simulink model "PMSM_Control_Using_FOC_And_SVPWM_Conference"  (R2023b)
(part 2 of 5)

  Bus Selector15/2 -> Scope23/2  "<SOC (%)>"
  Bus Selector15/3 -> Scope23/3  "<Current (A)>"
  Signal Builder/1(torque) -> PMSM AC  5/1
  Speed_Path/1(speed) -> Sum18/1
  PID Controller22/1 -> PWM Generator (DC-DC)6/1
  Speed_Path1/1(speed) -> Sum29/1
  Signal Builder2/1(torque) -> PMSM AC  8/1
  SVPWM Generator (2-Level)8/1 -> Universal Bridge8/1
  PID Controller27/1 -> Scope25/1, Sum28/1
  Current Measurement2/1 -> Scope27/1
  Voltage Measurement8/1 -> Display13/1
  Gain23/1 -> Scope24/1
  Demux15/3 -> Terminator14/1
  Bus Selector17/6 -> Scope24/2  "<Electromagnetic torque Te (N*m)>"
  PID Controller29/1 -> Mux15/2
  PMSM AC  8/1 -> Bus Selector17/1
  Bus Selector17/3 -> Scope24/6, Mux16/3  "<Stator current is_c (A)>"
  Gain22/1 -> Sum29/2
  Sum27/1 -> Scope25/2, PID Controller28/1
  Bus Selector17/1 -> Scope24/4, Mux16/1  "<Stator current is_a (A)>"
  Constant36/1 -> Mux15/3
  PID Controller28/1 -> Mux15/1
  Mux15/1 -> dq0 to Alpha-Beta-Zero7/1
  Sum28/1 -> PID Controller29/1
  Bus Selector17/4 -> Gain23/1, Gain22/1  "<Rotor speed wm (rad/s)>"
  Demux16/2 -> Sum28/2
  Demux16/1 -> Sum27/2
  Bus Selector17/5 -> Scope24/3, Gain21/1  "<Rotor angle thetam (rad)>"
  Alpha-Beta-Zero to dq7/1 -> Demux16/1
  dq0 to Alpha-Beta-Zero7/1 -> Demux15/1
  Gain21/1 -> Alpha-Beta-Zero to dq7/2, dq0 to Alpha-Beta-Zero7/2
  Demux15/1 -> SVPWM Generator (2-Level)8/1
  Demux16/3 -> Terminator15/1
  Demux15/2 -> SVPWM Generator (2-Level)8/2
  Bus Selector17/2 -> Scope24/5, Mux16/2  "<Stator current is_b (A)>"
  Sum29/1 -> PID Controller27/1
  Constant34/1 -> Sum27/1
  abc to Alpha-Beta-Zero7/1 -> Alpha-Beta-Zero to dq7/1
  Voltage Measurement9/1 -> Display17/1, Sum31/2
  PWM Generator (DC-DC)4/1 -> Switch/3, Scope29/1
  Battery11/1 -> Bus Selector18/1
  Bus Selector18/1 -> Scope31/1  "<SOC (%)>"
  Step16/1 -> Add5/4
  Bus Selector18/3 -> Scope31/3  "<Voltage (V)>"
  Bus Selector18/2 -> Scope31/2  "<Current (A)>"
  Step13/1 -> Add5/1
  Current Measurement3/1 -> Sum30/2
  Step15/1 -> Add5/3
  Step14/1 -> Add5/2
  Voltage Measurement12/1 -> Display18/1
  Mux16/1 -> abc to Alpha-Beta-Zero7/1
  Add5/1 -> Sum30/1
  Sum30/1 -> PID Controller30/1
  PID Controller30/1 -> PWM Generator (DC-DC)4/1
  PID Controller31/1 -> PWM Generator (DC-DC)5/1
  Constant37/1 -> Sum31/1
  PWM Generator (DC-DC)5/1 -> Switch/1
  Sum31/1 -> PID Controller31/1
  Switch/1 -> Mosfet4/1, NOT/1
  NOT/1 -> Mosfet5/1
  Constant35/1 -> Switch/2
  Demux18/1 -> Sum32/2
  Battery8/1 -> Bus Selector19/1
  Demux18/3 -> Terminator17/1
  abc to Alpha-Beta-Zero8/1 -> Alpha-Beta-Zero to dq8/1
  Bus Selector16/2 -> Scope26/5, Mux18/2  "<Stator current is_b (A)>"
  PMSM AC  9/1 -> Bus Selector16/1
  Bus Selector16/4 -> Gain26/1, Gain25/1  "<Rotor speed wm (rad/s)>"
  Sum34/1 -> PID Controller32/1
  Speed_Path2/1(speed) -> Sum34/1
  PID Controller36/1 -> PWM Generator (DC-DC)9/1
  Signal Builder1/1(torque) -> PMSM AC  9/1
  Voltage Measurement14/1 -> Display14/1
  PID Controller33/1 -> Mux17/1
  Bus Selector16/1 -> Scope26/4, Mux18/1  "<Stator current is_a (A)>"
  SVPWM Generator (2-Level)9/1 -> Universal Bridge9/1
  Gain24/1 -> Alpha-Beta-Zero to dq8/2, dq0 to Alpha-Beta-Zero8/2
  Bus Selector16/3 -> Scope26/6, Mux18/3  "<Stator current is_c (A)>"
  Sum32/1 -> Scope28/2, PID Controller33/1
  Current Measurement4/1 -> Scope30/1
  Demux17/2 -> SVPWM Generator (2-Level)9/2
  Sum36/1 -> PID Controller36/1
  PID Controller32/1 -> Scope28/1, Sum33/1
  Gain26/1 -> Scope26/1
  PID Controller34/1 -> Mux17/2
  Bus Selector19/1 -> Scope32/1, Scope33/1  "<SOC (%)>"
  Demux17/1 -> SVPWM Generator (2-Level)9/1
  Constant40/1 -> Mux17/3
  Bus Selector19/3 -> Scope33/3  "<Voltage (V)>"
  Alpha-Beta-Zero to dq8/1 -> Demux18/1
  Bus Selector16/6 -> Scope32/2, Scope26/2  "<Electromagnetic torque Te (N*m)>"
  PWM Generator (DC-DC)9/1 -> Mosfet8/1, NOT1/1
  Sum33/1 -> PID Controller34/1
  Demux17/3 -> Terminator16/1
  Gain25/1 -> Sum34/2
  Demux18/2 -> Sum33/2
  Constant38/1 -> Sum32/1
  Mux18/1 -> abc to Alpha-Beta-Zero8/1
  Mux17/1 -> dq0 to Alpha-Beta-Zero8/1
  Bus Selector19/2 -> Scope33/2  "<Current (A)>"
  Bus Selector16/5 -> Scope26/3, Gain24/1  "<Rotor angle thetam (rad)>"
  dq0 to Alpha-Beta-Zero8/1 -> Demux17/1
  Voltage Measurement13/1 -> Display20/1
  NOT1/1 -> Mosfet9/1
  Constant41/1 -> Sum36/1
  Voltage Measurement15/1 -> Display19/1, Sum36/2
  Voltage Measurement18/1 -> Sum39/2, Display22/1
  Constant43/1 -> Sum39/1
  NOT2/1 -> Mosfet11/1
  Voltage Measurement16/1 -> Display23/1
  dq0 to Alpha-Beta-Zero9/1 -> Demux19/1
  Bus Selector20/5 -> Gain27/1, Scope34/3  "<Rotor angle thetam (rad)>"
  Bus Selector21/2 -> Scope38/2  "<Current (A)>"
  Mux19/1 -> dq0 to Alpha-Beta-Zero9/1
  Mux20/1 -> abc to Alpha-Beta-Zero9/1
  Constant39/1 -> Sum35/1
  Demux20/2 -> Sum37/2
  Gain28/1 -> Sum38/2
  Demux19/3 -> Terminator18/1
  Sum37/1 -> PID Controller38/1
  PWM Generator (DC-DC)8/1 -> NOT2/1, Mosfet10/1
  Bus Selector20/6 -> Scope34/2, Scope37/2  "<Electromagnetic torque Te (N*m)>"
  Alpha-Beta-Zero to dq9/1 -> Demux20/1
  Bus Selector21/3 -> Scope38/3  "<Voltage (V)>"
  Constant42/1 -> Mux19/3
  Demux19/1 -> SVPWM Generator (2-Level)10/1
  Bus Selector21/1 -> Scope38/1, Scope37/1  "<SOC (%)>"
  PID Controller38/1 -> Mux19/2
  Gain29/1 -> Scope34/1
  PID Controller35/1 -> Sum37/1, Scope35/1
  Sum39/1 -> PID Controller39/1
  Demux19/2 -> SVPWM Generator (2-Level)10/2
  Current Measurement6/1 -> Scope36/1
  Sum35/1 -> PID Controller37/1, Scope35/2
  Bus Selector20/3 -> Mux20/3, Scope34/6  "<Stator current is_c (A)>"
  Gain27/1 -> dq0 to Alpha-Beta-Zero9/2, Alpha-Beta-Zero to dq9/2
  SVPWM Generator (2-Level)10/1 -> Universal Bridge10/1
  Bus Selector20/1 -> Mux20/1, Scope34/4  "<Stator current is_a (A)>"
  PID Controller37/1 -> Mux19/1
  Voltage Measurement17/1 -> Display21/1
  Sum38/1 -> PID Controller35/1
  Bus Selector20/4 -> Gain28/1, Gain29/1  "<Rotor speed wm (rad/s)>"
  PMSM AC  10/1 -> Bus Selector20/1
  Bus Selector20/2 -> Mux20/2, Scope34/5  "<Stator current is_b (A)>"
  abc to Alpha-Beta-Zero9/1 -> Alpha-Beta-Zero to dq9/1
  Demux20/3 -> Terminator19/1
  Battery12/1 -> Bus Selector21/1
  Demux20/1 -> Sum35/2
  Multiport Switch/1 -> PMSM AC  10/1
  Scenario_Selection/1 -> Multiport Switch/1, Multiport Switch1/1
  Multiport Switch1/1 -> Sum38/1
  Speed_Path6/1(speed) -> Multiport Switch1/2
  Signal Builder8/1(torque) -> Multiport Switch/3
  Speed_Path8/1(speed) -> Multiport Switch1/3
  Demux22/1 -> Sum40/2
  PID Controller42/1 -> Mux21/2
  Bus Selector23/1 -> Scope43/1, Scope42/1  "<SOC (%)>"
  Bus Selector22/1 -> Mux22/1, Scope39/4  "<Stator current is_a (A)>"
  Bus Selector23/3 -> Scope43/3  "<Voltage (V)>"
  Bus Selector22/4 -> Gain31/1, Gain32/1  "<Rotor speed wm (rad/s)>"
  Demux21/2 -> SVPWM Generator (2-Level)11/2
  Sum42/1 -> PID Controller40/1
  Bus Selector22/6 -> Scope39/2  "<Electromagnetic torque Te (N*m)>"
  Switch2/1 -> Sum42/1
  Constant45/1 -> Mux21/3
  Bus Selector22/2 -> Mux22/2, Scope39/5  "<Stator current is_b (A)>"
  Gain30/1 -> dq0 to Alpha-Beta-Zero10/2, Alpha-Beta-Zero to dq10/2
  Demux22/3 -> Terminator21/1
  Demux22/2 -> Sum41/2
  Demux21/3 -> Terminator20/1
  SVPWM Generator (2-Level)11/1 -> Universal Bridge11/1
  Switch1/1 -> PMSM AC  11/1
  Sum41/1 -> PID Controller42/1
  Mux22/1 -> abc to Alpha-Beta-Zero10/1
  Scenario_Selection1/1 -> Switch2/2, Switch1/2
  Current Measurement8/1 -> Scope41/1
  Speed_Path3/1(speed) -> Switch2/1
  Sum40/1 -> PID Controller41/1, Scope40/2
  PID Controller41/1 -> Mux21/1
  Battery13/1 -> Bus Selector23/1
  PMSM AC  11/1 -> Bus Selector22/1
  Speed_Path5/1(speed) -> Switch2/3
  Signal Builder5/1(torque) -> Switch1/3
  Signal Builder3/1(torque) -> Switch1/1
  Mux21/1 -> dq0 to Alpha-Beta-Zero10/1
  Voltage Measurement19/1 -> Display26/1
  Gain32/1 -> Scope39/1
  PID Controller40/1 -> Sum41/1, Scope40/1
  dq0 to Alpha-Beta-Zero10/1 -> Demux21/1
  Voltage Measurement20/1 -> Display24/1
  Voltage Measurement21/1 -> Scope42/3, Display25/1
  Alpha-Beta-Zero to dq10/1 -> Demux22/1
  Demux21/1 -> SVPWM Generator (2-Level)11/1
  Gain31/1 -> Sum42/2
  Bus Selector23/2 -> Scope42/2, Scope43/2  "<Current (A)>"
  Constant44/1 -> Sum40/1
  abc to Alpha-Beta-Zero10/1 -> Alpha-Beta-Zero to dq10/1
  Bus Selector22/5 -> Gain30/1, Scope39/3  "<Rotor angle thetam (rad)>"
  Bus Selector22/3 -> Mux22/3, Scope39/6  "<Stator current is_c (A)>"
  Bus Selector24/1 -> Scope46/1, Display27/1  "<Voltage (V)>"
  Constant47/1 -> Sum44/2
  Battery14/1 -> Bus Selector24/1
  Bus Selector24/2 -> Display31/1, Scope46/2  "<Current (A)>"
  Bus Selector24/3 -> Scope46/3  "<SOC (%)>"
  PWM Generator (DC-DC)11/1 -> NOT4/1, Scope47/1, PWM_1/1
  NOT4/1 -> Scope48/1, PWM_2/1
  Current Measurement10/1 -> Display30/1
  Voltage Measurement23/1 -> Sum44/1, Scope45/1, Display28/1
  Voltage Measurement22/1 -> Display29/1
  From1/1 -> Mosfet14/1
  PID Controller45/1 -> PWM Generator (DC-DC)11/1, Display32/1
  Sum44/1 -> PID Controller45/1
  Constant48/1 -> Sum45/1
  Sum45/1 -> Fuzzy Logic Controller1/1
  Fuzzy Logic Controller1/1 -> Display33/1, PWM Generator (DC-DC)12/1
  NOT5/1 -> PWM_4/1, Scope50/1
  PWM Generator (DC-DC)12/1 -> PWM_3/1, Scope49/1, NOT5/1
  From/1 -> Mosfet15/1
  Voltage Measurement24/1 -> Scope51/1
  PWM Generator (DC-DC)13/1 -> Mosfet12/1, NOT6/1
  Constant50/1 -> PWM Generator (DC-DC)13/1
  PWM Generator (DC-DC)14/1 -> Mosfet16/1, NOT7/1
  NOT7/1 -> Mosfet17/1
  Constant51/1 -> PWM Generator (DC-DC)14/1
  NOT6/1 -> Mosfet13/1
  PID Controller39/1 -> PWM Generator (DC-DC)8/1
  PWM Generator (DC-DC)2/1 -> Mosfet3/1
  PWM Generator (DC-DC)3/1 -> Mosfet2/1
  Bus Selector25/2 -> Scope52/2, Scope44/2  "<Current (A)>"
  Voltage Measurement25/1 -> Display37/1
  Battery15/1 -> Bus Selector25/1
  Bus Selector25/3 -> Goto2/1, Scope52/3  "<Voltage (V)>"
  Bus Selector25/1 -> Scope44/1, Goto1/1, Scope52/1, Goto/1  "<SOC (%)>"
  From2/1 -> Mosfet22/1
  From3/1 -> Mosfet23/1
  Voltage Measurement27/1 -> Display38/1, Goto3/1
  Sum43/1 -> PID Controller43/1
  Constant53/1 -> Sum43/1
  From4/1 -> Sum43/2
  PID Controller43/1 -> Goto4/1
  PID Controller44/1 -> Gain33/1
  From5/1 -> Sum46/2
  Constant54/1 -> Sum46/1
  Sum46/1 -> PID Controller44/1
  Gain33/1 -> Goto5/1
  From6/1 -> Switch3/1
  From7/1 -> Switch3/3
  From8/1 -> Switch3/2
  Step10/1 -> Goto6/1
  From9/1 -> Ideal Switch/1
  From10/1 -> Sum47/2
  From11/1 -> Sum47/1
  Sum47/1 -> PID Controller46/1
  Switch3/1 -> Goto8/1
  PID Controller46/1 -> PWM Generator (DC-DC)16/1
  PWM Generator (DC-DC)16/1 -> NOT9/1, Goto7/1
  NOT9/1 -> Goto9/1
  From13/1 -> Mosfet19/1
  From12/1 -> Mosfet18/1
  Bus Selector26/1 -> Goto10/1, Scope54/1, Goto11/1, Scope53/1  "<SOC (%)>"
  Bus Selector26/3 -> Scope54/3, Goto12/1  "<Voltage (V)>"
  Bus Selector26/2 -> Scope53/2, Scope54/2  "<Current (A)>"
  Battery16/1 -> Bus Selector26/1
  Current Measurement9/1 -> Display40/1, Goto13/1
  NOT3/1 -> Goto15/1
  PWM Generator (DC-DC)10/1 -> Goto14/1, NOT3/1
  PID Controller47/1 -> Display41/1, PWM Generator (DC-DC)10/1
  Sum48/1 -> PID Controller47/1
  Constant46/1 -> Sum48/1
  From14/1 -> Sum48/2
  Voltage Measurement26/1 -> Display36/1
  Voltage Measurement28/1 -> Display39/1
  Signal Builder11/1(torque) -> Multiport Switch/2
  Torque_Input/1(torque) -> "PMSM AC "/1, To Workspace8/1
  "Battery "/1 -> Bus Selector28/1
  Bus Selector27/2 -> Field-Oriented Control/4(<Stator current is_b (A)>), Scope55/5  "<Stator current is_b (A)>"
  "PMSM AC "/1 -> Bus Selector27/1
  Bus Selector27/4 -> Field-Oriented Control/3(<Rotor speed wm (rad/s)>), Gain36/1  "<Rotor speed wm (rad/s)>"
  Bus Selector27/1 -> Scope55/4, Field-Oriented Control/2(<Stator current is_a (A)>)  "<Stator current is_a (A)>"
  Bus Selector27/3 -> Field-Oriented Control/5(<Stator current is_c (A)>), Scope55/6  "<Stator current is_c (A)>"
  Gain36/1 -> To Workspace4/1, Scope55/1
  Bus Selector28/1 -> Scope59/1, To Workspace/1  "<SOC (%)>"
  Bus Selector28/3 -> Scope59/3  "<Voltage (V)>"
  Bus Selector27/6 -> To Workspace5/1, Scope55/2  "<Electromagnetic torque Te (N*m)>"
  Bus Selector28/2 -> Scope59/2  "<Current (A)>"
  Bus Selector27/5 -> Field-Oriented Control/6(<Rotor angle thetam (rad)>), Scope55/3  "<Rotor angle thetam (rad)>"
  Speed_Ref/1(speed) -> To Workspace9/1, Field-Oriented Control/1(Speed_Ref)
  Field-Oriented Control/1(Gates) -> Full_Bridge/1(g)
  PMSM AC/1 -> Bus Selector31/1
  Bus Selector31/2 -> Subsystem1/4(<Stator current is_b (A)>), Scope56/5  "<Stator current is_b (A)>"
  Bus Selector32/2 -> Scope57/2  "<Current (A)>"
  Bus Selector31/4 -> Subsystem1/3(<Rotor speed wm (rad/s)>), Gain34/1  "<Rotor speed wm (rad/s)>"
  Bus Selector31/5 -> Subsystem1/6(<Rotor angle thetam (rad)>), Scope56/3  "<Rotor angle thetam (rad)>"
  Bus Selector31/6 -> To Workspace7/1, Scope56/2  "<Electromagnetic torque Te (N*m)>"
  Gain34/1 -> To Workspace6/1, Scope56/1
  Battery19/1 -> Bus Selector32/1
  Recovered_Energy_Calculation/1(Output) -> To Workspace2/1, Display42/1
  Torque_Input1/1(torque) -> PMSM AC/1
  Subsystem1/1(Gates) -> "Full_Bridge "/1(g)
  Bus Selector31/3 -> Subsystem1/5(<Stator current is_c (A)>), Scope56/6  "<Stator current is_c (A)>"
  Speed_Ref1/1(speed) -> Subsystem1/1(Speed_Ref)
  Bus Selector32/3 -> Scope57/3  "<Voltage (V)>"
  Bus Selector32/1 -> Scope57/1, To Workspace1/1  "<SOC (%)>"
  Bus Selector31/1 -> Scope56/4, Subsystem1/2(<Stator current is_a (A)>)  "<Stator current is_a (A)>"
  Demux26/3 -> Terminator25/1
  Alpha-Beta-Zero to dq12/1 -> Demux26/1
  Sum55/1 -> PID Controller52/1
  SVPWM Generator (2-Level)13/1 -> Universal Bridge13/1
  Bus Selector30/3 -> Scope64/3  "<Voltage (V)>"
  Sum53/1 -> Scope61/2, PID Controller53/1
  Speed_Path12/1(speed) -> Sum55/1
  Constant58/1 -> Mux25/3
  dq0 to Alpha-Beta-Zero12/1 -> Demux25/1
  PID Controller52/1 -> Scope61/1, Sum54/1
  Gain38/1 -> Sum55/2
  Bus Selector29/2 -> Scope60/5, Mux26/2  "<Stator current is_b (A)>"
  PID Controller54/1 -> Mux25/2
  Gain37/1 -> Alpha-Beta-Zero to dq12/2, dq0 to Alpha-Beta-Zero12/2
  Current Measurement13/1 -> Scope62/1, Switch4/3, Product/2
  Bus Selector30/1 -> Scope64/1  "<SOC (%)>"
  Battery18/1 -> Bus Selector30/1
  Sum54/1 -> PID Controller54/1
  Bus Selector29/6 -> Scope60/2  "<Electromagnetic torque Te (N*m)>"
  Demux25/2 -> SVPWM Generator (2-Level)13/2
  Integrator/1 -> J to Wh/1
  Demux25/3 -> Terminator24/1
  Voltage Measurement33/1 -> Product/1, Display45/1
  Bus Selector29/5 -> Scope60/3, Gain37/1  "<Rotor angle thetam (rad)>"
  Switch4/1 -> Integrator/1
  Constant59/1 -> Switch4/1
  Bus Selector30/2 -> Scope64/2  "<Current (A)>"
  Gain39/1 -> Scope60/1
  Constant57/1 -> Sum53/1
  Demux25/1 -> SVPWM Generator (2-Level)13/1
  PID Controller53/1 -> Mux25/1
  Demux26/1 -> Sum53/2
  Signal Builder13/1(torque) -> PMSM AC  13/1
  PMSM AC  13/1 -> Bus Selector29/1
  Demux26/2 -> Sum54/2
  Bus Selector29/1 -> Scope60/4, Mux26/1  "<Stator current is_a (A)>"
  abc to Alpha-Beta-Zero12/1 -> Alpha-Beta-Zero to dq12/1
  Mux25/1 -> dq0 to Alpha-Beta-Zero12/1
  Bus Selector29/4 -> Gain39/1, Gain38/1  "<Rotor speed wm (rad/s)>"
  Mux26/1 -> abc to Alpha-Beta-Zero12/1
  Bus Selector29/3 -> Scope60/6, Mux26/3  "<Stator current is_c (A)>"
  Product/1 -> Switch4/2
  J to Wh/1 -> Display46/1, Scope63/1
  "Recovered_Energy_Calculation "/1(Output) -> To Workspace3/1, Display44/1
  Voltage Measurement32/1 -> Display47/1
  Voltage Measurement31/1 -> Display43/1
  Current Measurement14/1 -> Scope58/1
  Constant52/1 -> PWM Generator (DC-DC)15/1
  PWM Generator (DC-DC)15/1 -> NOT8/1, Mosfet20/1
  NOT8/1 -> Mosfet21/1
  Voltage Measurement34/1 -> Display48/1
  Battery20/1 -> Bus Selector33/1
  Bus Selector33/1 -> Display49/1  "<SOC (%)>"
  Bus Selector33/2 -> Display50/1  "<Current (A)>"
  Bus Selector33/3 -> Display51/1  "<Voltage (V)>"
  Voltage Measurement35/1 -> Recovered_Energy_Calculation_1/2(In2)
  Current Measurement15/1 -> Recovered_Energy_Calculation_1/1(In1)
  Recovered_Energy_Calculation_1/1(Output) -> Display52/1
  Field-Oriented Control1/1(Gates) -> Full_Bridge2/1(g)
  Speed_Ref2/1(speed) -> Field-Oriented Control1/1(Speed_Ref)
  Bus Selector34/5 -> Scope65/3, Field-Oriented Control1/6(<Rotor angle thetam (rad)>)  "<Rotor angle thetam (rad)>"
  Bus Selector35/2 -> Scope66/2  "<Current (A)>"
  Bus Selector34/6 -> Scope65/2  "<Electromagnetic torque Te (N*m)>"
  Bus Selector35/3 -> Scope66/3  "<Voltage (V)>"
  Bus Selector35/1 -> Scope66/1  "<SOC (%)>"
  Gain35/1 -> Scope65/1
  Bus Selector34/3 -> Scope65/6, Field-Oriented Control1/5(<Stator current is_c (A)>)  "<Stator current is_c (A)>"
  Bus Selector34/1 -> Field-Oriented Control1/2(<Stator current is_a (A)>), Scope65/4  "<Stator current is_a (A)>"
  Bus Selector34/4 -> Gain35/1, Field-Oriented Control1/3(<Rotor speed wm (rad/s)>)  "<Rotor speed wm (rad/s)>"
  PMSM AC  15/1 -> Bus Selector34/1
  Bus Selector34/2 -> Scope65/5, Field-Oriented Control1/4(<Stator current is_b (A)>)  "<Stator current is_b (A)>"
  Battery21/1 -> Bus Selector35/1
  Torque_Input2/1(torque) -> PMSM AC  15/1
  Constant55/1 -> DC Machine/1
  Current Measurement11/1 -> Recovered_Energy_Calculation/1(In1)
  Voltage Measurement29/1 -> Recovered_Energy_Calculation/2(In2)
  Voltage Measurement36/1 -> Display53/1, Scope67/1
  Voltage Measurement30/1 -> Scope68/1, Recovered_Energy_Calculation 1/2(In2), Recovered_Energy_Calculation 2/2(In2), "Recovered_Energy_Calculation "/2(In2)
  Recovered_Energy_Calculation 1/1(Output) -> Display54/1
  Current Measurement12/1 -> Recovered_Energy_Calculation 2/1(In1), Recovered_Energy_Calculation 1/1(In1), Scope69/1, "Recovered_Energy_Calculation "/1(In1)
  Recovered_Energy_Calculation 2/1(Output) -> Display55/1
  Recovered_Energy_Calculation 5/1(Output) -> Display58/1
  Recovered_Energy_Calculation 4/1(Output) -> Display57/1
  Recovered_Energy_Calculation 3/1(Output) -> To Workspace11/1, Display56/1
  Voltage Measurement37/1 -> Scope74/2, Scope72/1, Recovered_Energy_Calculation 4/2(In2), Recovered_Energy_Calculation 5/2(In2), Recovered_Energy_Calculation 3/2(In2)
  Bus Selector36/6 -> To Workspace13/1, Scope70/2  "<Electromagnetic torque Te (N*m)>"
  Torque_Input3/1(torque) -> PMSM AC 1/1, To Workspace14/1
  Gain40/1 -> To Workspace12/1, Scope70/1
  Bus Selector36/1 -> Scope70/4, Field-Oriented Control2/2(<Stator current is_a (A)>)  "<Stator current is_a (A)>"
  Bus Selector36/2 -> Field-Oriented Control2/4(<Stator current is_b (A)>), Scope70/5  "<Stator current is_b (A)>"
  Bus Selector36/3 -> Field-Oriented Control2/5(<Stator current is_c (A)>), Scope70/6  "<Stator current is_c (A)>"
  Bus Selector37/1 -> Scope71/1, To Workspace10/1  "<SOC (%)>"
  Battery 1/1 -> Bus Selector37/1
  Field-Oriented Control2/1(Gates) -> Full_Bridge1/1(g)
  Bus Selector36/4 -> Field-Oriented Control2/3(<Rotor speed wm (rad/s)>), Gain40/1  "<Rotor speed wm (rad/s)>"
  Bus Selector37/3 -> Scope71/3  "<Voltage (V)>"
  Bus Selector37/2 -> Scope71/2  "<Current (A)>"
  Bus Selector36/5 -> Field-Oriented Control2/6(<Rotor angle thetam (rad)>), Scope70/3  "<Rotor angle thetam (rad)>"
  PMSM AC 1/1 -> Bus Selector36/1
  Speed_Ref3/1(speed) -> To Workspace15/1, Field-Oriented Control2/1(Speed_Ref)
  Current Measurement16/1 -> Recovered_Energy_Calculation 5/1(In1), Recovered_Energy_Calculation 4/1(In1), Scope73/1, Recovered_Energy_Calculation 3/1(In1)
  Voltage Measurement38/1 -> Scope74/1
  connections:
  DC Voltage5/LConn1 -- Universal Bridge5/RConn2
  DC Voltage5/RConn1 -- Universal Bridge5/RConn1
  Universal Bridge5/LConn1 -- PMSM AC  2/LConn1
  Universal Bridge5/LConn2 -- PMSM AC  2/LConn2
  Universal Bridge5/LConn3 -- PMSM AC  2/LConn3
  Series RLC Branch1/RConn1 -- Voltage Measurement/LConn1 -- Battery1/LConn1 -- Series RLC Branch/LConn1
  Series RLC Branch1/LConn1 -- Mosfet/LConn1 -- Mosfet1/RConn1
  Series RLC Branch/RConn1 -- Battery1/LConn2 -- Voltage Measurement/LConn2 -- Battery2/LConn2 -- Voltage Measurement1/LConn2 -- Series RLC Branch2/RConn1 -- Mosfet/RConn1
  Series RLC Branch2/LConn1 -- Battery2/LConn1 -- Voltage Measurement1/LConn1 -- Mosfet1/LConn1
  Universal Bridge1/LConn2 -- Three-Phase V-I Measurement/LConn2
  Voltage Measurement2/LConn1 -- Current Measurement/RConn1 -- Universal Bridge1/RConn1
  Universal Bridge1/LConn1 -- Three-Phase V-I Measurement/LConn1
  Voltage Measurement2/LConn2 -- Battery3/LConn2 -- Universal Bridge1/RConn2
  Universal Bridge1/LConn3 -- Three-Phase V-I Measurement/LConn3
  Mosfet2/RConn1 -- Battery5/LConn2 -- Voltage Measurement4/LConn2 -- Series RLC Branch3/RConn1 -- Universal Bridge2/RConn2 -- Voltage Measurement3/LConn2 -- Voltage Measurement5/LConn2 -- Series RLC Branch5/RConn1
  Universal Bridge2/LConn3 -- PMSM AC  3/LConn3
  Universal Bridge2/LConn1 -- PMSM AC  3/LConn1
  Universal Bridge2/LConn2 -- PMSM AC  3/LConn2
  Series RLC Branch4/RConn1 -- Voltage Measurement4/LConn1 -- Battery5/LConn1 -- Series RLC Branch3/LConn1
  Series RLC Branch4/LConn1 -- Mosfet3/LConn1 -- Mosfet2/LConn1
  Voltage Measurement3/LConn1 -- Mosfet3/RConn1 -- Series RLC Branch5/LConn1 -- Voltage Measurement5/LConn1 -- Universal Bridge2/RConn1
  Current Measurement/LConn1 -- Battery3/LConn1
  Three-Phase V-I Measurement/RConn1 -- PMSM AC  1/LConn1
  Three-Phase V-I Measurement/RConn2 -- PMSM AC  1/LConn2
  Three-Phase V-I Measurement/RConn3 -- PMSM AC  1/LConn3
  Voltage Measurement6/LConn2 -- Universal Bridge3/RConn2 -- Battery4/LConn2
  Voltage Measurement6/LConn1 -- Battery4/LConn1 -- Universal Bridge3/RConn1
  Universal Bridge3/LConn3 -- PMSM AC  4/LConn3
  Universal Bridge3/LConn2 -- PMSM AC  4/LConn2
  Universal Bridge3/LConn1 -- PMSM AC  4/LConn1
  Universal Bridge4/LConn2 -- PMSM AC  5/LConn2
  Universal Bridge4/LConn1 -- PMSM AC  5/LConn1
  Universal Bridge4/RConn2 -- Battery6/LConn2 -- Series RLC Branch6/RConn1 -- Voltage Measurement7/LConn2
  Universal Bridge4/LConn3 -- PMSM AC  5/LConn3
  Voltage Measurement7/LConn1 -- Current Measurement1/RConn1 -- Universal Bridge4/RConn1
  Current Measurement1/LConn1 -- Battery6/LConn1 -- Series RLC Branch6/LConn1
  Series RLC Branch7/RConn1 -- Battery9/LConn2 -- Voltage Measurement10/LConn2 -- Series RLC Branch11/RConn1 -- Battery10/LConn2 -- Voltage Measurement11/LConn2 -- Mosfet6/RConn1
  Voltage Measurement11/LConn1 -- Battery10/LConn1 -- Series RLC Branch11/LConn1 -- Mosfet7/LConn1
  Series RLC Branch10/LConn1 -- Mosfet7/RConn1 -- Mosfet6/LConn1
  Series RLC Branch7/LConn1 -- Series RLC Branch10/RConn1 -- Voltage Measurement10/LConn1 -- Battery9/LConn1
  Universal Bridge6/LConn2 -- PMSM AC  6/LConn2
  Universal Bridge6/LConn1 -- PMSM AC  6/LConn1
  DC Voltage1/LConn1 -- Universal Bridge6/RConn2
  Universal Bridge6/LConn3 -- PMSM AC  6/LConn3
  DC Voltage1/RConn1 -- Universal Bridge6/RConn1
  Universal Bridge7/LConn2 -- PMSM AC  7/LConn2
  Universal Bridge7/LConn1 -- PMSM AC  7/LConn1
  Universal Bridge7/RConn2 -- Battery7/LConn2 -- Series RLC Branch8/RConn1
  Universal Bridge7/LConn3 -- PMSM AC  7/LConn3
  Universal Bridge7/RConn1 -- Battery7/LConn1 -- Series RLC Branch8/LConn1
  Voltage Measurement12/LConn2 -- Mosfet5/RConn1 -- Series RLC Branch9/RConn1 -- Voltage Measurement8/LConn2 -- Universal Bridge8/RConn2 -- Voltage Measurement9/LConn2 -- Series RLC Branch14/RConn1 -- Battery11/LConn2
  Voltage Measurement8/LConn1 -- Current Measurement2/RConn1 -- Universal Bridge8/RConn1
  Universal Bridge8/LConn2 -- PMSM AC  8/LConn2
  Universal Bridge8/LConn1 -- PMSM AC  8/LConn1
  Universal Bridge8/LConn3 -- PMSM AC  8/LConn3
  Mosfet4/RConn1 -- Series RLC Branch12/LConn1 -- Mosfet5/LConn1
  Voltage Measurement12/LConn1 -- Battery11/LConn1 -- Series RLC Branch14/LConn1 -- Mosfet4/LConn1
  Voltage Measurement9/LConn1 -- Current Measurement2/LConn1 -- Series RLC Branch9/LConn1 -- Current Measurement3/RConn1
  Current Measurement3/LConn1 -- Series RLC Branch12/RConn1
  Current Measurement5/RConn1 -- Voltage Measurement15/LConn1 -- Current Measurement4/LConn1 -- Series RLC Branch16/LConn1
  Universal Bridge9/RConn2 -- Mosfet9/RConn1 -- Voltage Measurement13/LConn2 -- Battery8/LConn2 -- Series RLC Branch15/RConn1 -- Voltage Measurement15/LConn2 -- Series RLC Branch16/RConn1 -- Voltage Measurement14/LConn2
  Mosfet8/LConn1 -- Voltage Measurement13/LConn1 -- Battery8/LConn1 -- Series RLC Branch15/LConn1
  Universal Bridge9/RConn1 -- Current Measurement4/RConn1 -- Voltage Measurement14/LConn1
  Mosfet9/LConn1 -- Mosfet8/RConn1 -- Series RLC Branch13/LConn1
  Universal Bridge9/LConn2 -- PMSM AC  9/LConn2
  Universal Bridge9/LConn1 -- PMSM AC  9/LConn1
  Universal Bridge9/LConn3 -- PMSM AC  9/LConn3
  Current Measurement5/LConn1 -- Series RLC Branch13/RConn1
  Current Measurement7/RConn1 -- Series RLC Branch19/LConn1 -- Current Measurement6/LConn1 -- Voltage Measurement18/LConn1
  Universal Bridge10/RConn2 -- Voltage Measurement17/LConn2 -- Series RLC Branch19/RConn1 -- Voltage Measurement18/LConn2 -- Series RLC Branch18/RConn1 -- Battery12/LConn2 -- Voltage Measurement16/LConn2 -- Mosfet11/RConn1
  Mosfet10/LConn1 -- Series RLC Branch18/LConn1 -- Battery12/LConn1 -- Voltage Measurement16/LConn1
  Universal Bridge10/RConn1 -- Voltage Measurement17/LConn1 -- Current Measurement6/RConn1
  Mosfet11/LConn1 -- Series RLC Branch17/LConn1 -- Mosfet10/RConn1
  Universal Bridge10/LConn3 -- PMSM AC  10/LConn3
  Universal Bridge10/LConn1 -- PMSM AC  10/LConn1
  Universal Bridge10/LConn2 -- PMSM AC  10/LConn2
  Current Measurement7/LConn1 -- Series RLC Branch17/RConn1
  Voltage Measurement19/LConn2 -- Series RLC Branch21/RConn1 -- Battery13/LConn2 -- Mosfet17/RConn1 -- Series RLC Branch27/RConn1 -- Series RLC Branch22/RConn1 -- Voltage Measurement21/LConn2 -- Mosfet13/RConn1
  Universal Bridge11/LConn1 -- PMSM AC  11/LConn1
  Universal Bridge11/LConn3 -- PMSM AC  11/LConn3
  Universal Bridge11/LConn2 -- PMSM AC  11/LConn2
  Voltage Measurement22/LConn1 -- Battery14/LConn1 -- Current Measurement10/RConn1
  Voltage Measurement23/LConn1 -- Series RLC Branch26/LConn1 -- Mosfet15/LConn1 -- Series RLC Branch25/LConn1
  Series RLC Branch23/RConn1 -- Voltage Measurement22/LConn2 -- Battery14/LConn2 -- Voltage Measurement24/LConn2 -- Series RLC Branch26/RConn1 -- Voltage Measurement23/LConn2 -- Series RLC Branch25/RConn1 -- Mosfet14/RConn1
  Universal Bridge11/RConn1 -- Current Measurement8/RConn1 -- Voltage Measurement20/LConn1
  Series RLC Branch24/RConn1 -- Current Measurement10/LConn1 -- Series RLC Branch23/LConn1
  Voltage Measurement20/LConn2 -- Universal Bridge11/RConn2
  Series RLC Branch24/LConn1 -- Voltage Measurement24/LConn1 -- Mosfet14/LConn1 -- Mosfet15/RConn1
  Mosfet13/LConn1 -- Mosfet12/RConn1 -- Series RLC Branch20/RConn1
  Mosfet17/LConn1 -- Mosfet16/RConn1 -- Series RLC Branch20/LConn1
  Series RLC Branch21/LConn1 -- Voltage Measurement19/LConn1 -- Battery13/LConn1 -- Mosfet16/LConn1
  Voltage Measurement21/LConn1 -- Series RLC Branch27/LConn1 -- Series RLC Branch22/LConn1 -- Mosfet12/LConn1
  Battery15/LConn1 -- Series RLC Branch33/LConn1 -- Series RLC Branch32/LConn1 -- Voltage Measurement25/LConn1
  Series RLC Branch32/RConn1 -- Voltage Measurement27/LConn2 -- Series RLC Branch34/RConn1 -- DC Voltage Source/LConn1 -- Mosfet23/RConn1 -- Voltage Measurement25/LConn2 -- Battery15/LConn2
  Mosfet22/RConn1 -- Mosfet23/LConn1 -- Series RLC Branch33/RConn1
  Ideal Switch/RConn1 -- Voltage Measurement27/LConn1 -- Series RLC Branch34/LConn1 -- Mosfet22/LConn1
  DC Voltage Source/RConn1 -- Ideal Switch/LConn1
  Series RLC Branch29/LConn1 -- Current Measurement9/LConn1 -- Series RLC Branch28/LConn1
  Series RLC Branch30/RConn1 -- Voltage Measurement26/LConn2 -- Mosfet19/RConn1 -- Voltage Measurement28/LConn2 -- Battery16/LConn2 -- Series RLC Branch28/RConn1 -- Series RLC Branch31/RConn1
  Mosfet19/LConn1 -- Mosfet18/RConn1 -- Series RLC Branch29/RConn1
  Series RLC Branch30/LConn1 -- Voltage Measurement26/LConn1 -- Series RLC Branch31/LConn1 -- Mosfet18/LConn1
  Current Measurement9/RConn1 -- Voltage Measurement28/LConn1 -- Battery16/LConn1
  Full_Bridge/LConn1 -- "PMSM AC "/LConn1
  Full_Bridge/LConn2 -- "PMSM AC "/LConn2
  Full_Bridge/LConn3 -- "PMSM AC "/LConn3
  Bidirectional_Converter/RConn1 -- Full_Bridge/RConn1
  Bidirectional_Converter/RConn2 -- Full_Bridge/RConn2
  Voltage Measurement29/LConn2 -- Unidirectional_Converter/LConn2 -- Battery19/LConn2
  Battery19/LConn1 -- Voltage Measurement29/LConn1 -- Current Measurement11/LConn1
  "Full_Bridge "/LConn1 -- PMSM AC/LConn1
  "Full_Bridge "/LConn3 -- PMSM AC/LConn3
  "Full_Bridge "/LConn2 -- PMSM AC/LConn2
  Universal Bridge13/RConn2 -- Series RLC Branch38/RConn1 -- Voltage Measurement33/LConn2 -- Battery18/LConn2
  Current Measurement13/RConn1 -- Series RLC Branch38/LConn1 -- Universal Bridge13/RConn1
  Battery18/LConn1 -- Current Measurement13/LConn1 -- Voltage Measurement33/LConn1
  Universal Bridge13/LConn1 -- PMSM AC  13/LConn1
  Universal Bridge13/LConn3 -- PMSM AC  13/LConn3
  Universal Bridge13/LConn2 -- PMSM AC  13/LConn2
  Current Measurement12/LConn1 -- "Battery "/LConn1 -- Voltage Measurement30/LConn1
  Voltage Measurement30/LConn2 -- Bidirectional_Converter/LConn2 -- "Battery "/LConn2
  Current Measurement12/RConn1 -- Bidirectional_Converter/LConn1
  Current Measurement14/LConn1 -- Series RLC Branch37/LConn1 -- Voltage Measurement32/LConn1 -- Mosfet20/LConn1
  Mosfet20/RConn1 -- Series RLC Branch35/RConn1 -- Mosfet21/LConn1
  Series RLC Branch36/LConn1 -- Voltage Measurement34/LConn1 -- Battery20/LConn1 -- Series RLC Branch35/LConn1
  Voltage Measurement31/LConn1 -- DC Machine/RConn1 -- Current Measurement14/RConn1
  Series RLC Branch36/RConn1 -- Voltage Measurement34/LConn2 -- Battery20/LConn2 -- Mosfet21/RConn1 -- Voltage Measurement31/LConn2 -- DC Machine/LConn1 -- Series RLC Branch37/RConn1 -- Voltage Measurement32/LConn2
  Current Measurement15/LConn1 -- Voltage Measurement35/LConn1 -- Battery21/LConn1
  Voltage Measurement35/LConn2 -- Battery21/LConn2 -- Bidirectional_Converter1/LConn2
  Full_Bridge2/LConn1 -- PMSM AC  15/LConn1
  Full_Bridge2/LConn2 -- PMSM AC  15/LConn2
  Full_Bridge2/LConn3 -- PMSM AC  15/LConn3
  Bidirectional_Converter1/RConn1 -- Full_Bridge2/RConn1
  Bidirectional_Converter1/RConn2 -- Full_Bridge2/RConn2
  Current Measurement15/RConn1 -- Bidirectional_Converter1/LConn1
  Unidirectional_Converter/RConn1 -- Voltage Measurement36/LConn1 -- "Full_Bridge "/RConn1
  Unidirectional_Converter/RConn2 -- Voltage Measurement36/LConn2 -- "Full_Bridge "/RConn2
  Current Measurement11/RConn1 -- Unidirectional_Converter/LConn1
  Battery 1/LConn2 -- Voltage Measurement37/LConn2 -- Bidirectional_Converter3/LConn2
  Voltage Measurement37/LConn1 -- Current Measurement16/LConn1 -- Battery 1/LConn1
  Full_Bridge1/LConn2 -- PMSM AC 1/LConn2
  Bidirectional_Converter3/RConn1 -- Voltage Measurement38/LConn1 -- Full_Bridge1/RConn1
  Full_Bridge1/LConn1 -- PMSM AC 1/LConn1
  Full_Bridge1/LConn3 -- PMSM AC 1/LConn3
  Current Measurement16/RConn1 -- Bidirectional_Converter3/LConn1
  Bidirectional_Converter3/RConn2 -- Voltage Measurement38/LConn2 -- Full_Bridge1/RConn2
